simulink library "xbsStateMachine_r2"  (Simulink 5.0)
undefined symbols (not defined in the file or in its folder): xlDistRamDepth, xlMatrixToOutputVec, xlMatrixToStateInitVec, xlNumMealyElements, xlNumMooreOutputElements, xlNumMooreStateElements, xlNumStateBits, xlRegMealyInitVec
libraries: xbsMemory_r2 x7, xbsBasic_r2 x6
settings Model: Creator=administrator  LastModifiedBy=mcmillan

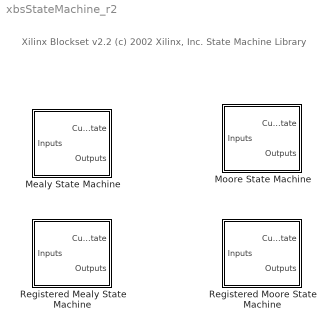
== system xbsStateMachine_r2 ==
  note: Xilinx Blockset v2.2
      | (c) 2002 Xilinx, Inc.
      |
      | State Machine Library
  Mealy State Machine : Subsystem  mask(Xilinx Mealy State Machine){next_state_matrix=[0 1; 2 1; 0 3; 2 1], output_matrix=[0 0; 0 0; 0 0; 0 1], n_bits=1, period=1, xl_area=[0, 0, 0, 0, 0, 0, 0], xl_use_area=off}
      mask prompts: next_state_matrix "Next State Matrix"; output_matrix "Output Matrix"; n_bits "Number of  Output Bits"; period "Sample Period"; xl_area "FPGA Area [Slices, FFs, BRAMs, LUTs, IOBs, Emb. Mults, TBUFs]"; xl_use_area "Use Area Above For Estimation"
      mask help: Implements a Mealy state machine. The output is a function of the current state and input.
      mask init:
      | % Set Block Logo
      | [bg,fg] = xlcmap('XBlock',0);
      | iPos = get_param(gcb,'Position');
      | iWidth=iPos(3)-iPos(1); iHeight=iPos(4)-iPos(2);
      | iCx=iWidth/2;
      | iCy=iHeight/2;
      | [logoX, logoY] = xlogo(iPos);
      mask Help: web(xldoclink('Mealy State Machine'));
      mask Display:
      | patch([0 iWidth iWidth 0],[0 0 iHeight iHeight] , bg);
      | patch(logoX,logoY, fg);
      | port_label('input',1,'Inputs');
      | port_label('output',1,'CurrentState');
      | port_label('output',2,'Outputs');
      | 
      | plot([0 0 iWidth iWidth 0], [0 iHeight iHeight 0 0]);
  Moore State Machine : Subsystem  mask(Xilinx Moore State Machine){next_state_matrix=[0 1; 2 1; 0 3; 2 4; 0 1], output_matrix=[0; 0; 0; 0; 1], n_bits=1, period=1, xl_area=[0, 0, 0, 0, 0, 0, 0], xl_use_area=off}
      mask prompts: next_state_matrix "Next State Matrix"; output_matrix "Output Array"; n_bits "Number of Output Bits"; period "Sample Period"; xl_area "FPGA Area [Slices, FFs, BRAMs, LUTs, IOBs, Emb. Mults, TBUFs]"; xl_use_area "Use Area Above For Estimation"
      mask help: Implements a Moore state machine. The output is a function only of the current state.
      mask init:
      | % Set Block Logo
      | [bg,fg] = xlcmap('XBlock',0);
      | iPos = get_param(gcb,'Position');
      | iWidth=iPos(3)-iPos(1); iHeight=iPos(4)-iPos(2);
      | iCx=iWidth/2;
      | iCy=iHeight/2;
      | [logoX, logoY] = xlogo(iPos);
      mask Help: web(xldoclink('Moore State Machine'));
      mask Display:
      | patch([0 iWidth iWidth 0],[0 0 iHeight iHeight] , bg);
      | patch(logoX,logoY, fg);
      | port_label('input',1,'Inputs');
      | port_label('output',1,'CurrentState');
      | port_label('output',2,'Outputs');
      | 
      | plot([0 0 iWidth iWidth 0], [0 iHeight iHeight 0 0]);
  Registered Mealy State Machine : Subsystem  mask(Xilinx Registered Mealy State Machine){next_state_matrix=[0 1; 2 1; 0 3; 2 1], output_matrix=[0 0; 0 0; 0 0; 0 1], n_bits=1, period=1, xl_area=[0, 0, 0, 0, 0, 0, 0], xl_use_area=off}
      mask prompts: next_state_matrix "Next State Matrix"; output_matrix "Output Matrix"; n_bits "Number of Output Bits"; period "Sample Period"; xl_area "FPGA Area [Slices, FFs, BRAMs, LUTs, IOBs, Emb. Mults, TBUFs]"; xl_use_area "Use Area Above For Estimation"
      mask help: Implements a registered Mealy state machine. The output is a function of the current state and its input. The output is registered.
      mask init:
      | % Set Block Logo
      | [bg,fg] = xlcmap('XBlock',0);
      | iPos = get_param(gcb,'Position');
      | iWidth=iPos(3)-iPos(1); iHeight=iPos(4)-iPos(2);
      | iCx=iWidth/2;
      | iCy=iHeight/2;
      | [logoX, logoY] = xlogo(iPos);
      mask Help: web(xldoclink('Registered Mealy State Machine'));
      mask Display:
      | patch([0 iWidth iWidth 0],[0 0 iHeight iHeight] , bg);
      | patch(logoX,logoY, fg);
      | port_label('input',1,'Inputs');
      | port_label('output',1,'CurrentState');
      | port_label('output',2,'Outputs');
      | 
      | plot([0 0 iWidth iWidth 0], [0 iHeight iHeight 0 0]);
  Registered Moore State Machine : Subsystem  mask(Xilinx Registered Moore State Machine){next_state_matrix=[0 1; 2 1; 0 3; 2 4; 0 1], output_matrix=[0; 0; 0; 0; 1], n_bits=1, period=1, xl_area=[0, 0, 0, 0, 0, 0, 0], xl_use_area=off}
      mask prompts: next_state_matrix "Next State Matrix"; output_matrix "Output Array"; n_bits "Number of Output Bits"; period "Sample Period"; xl_area "FPGA Area [Slices, FFs, BRAMs, LUTs, IOBs, Emb. Mults, TBUFs]"; xl_use_area "Use Area Above For Estimation"
      mask help: Implements a registered Moore state machine. The output is a function only of the current state. The output is registered.
      mask init:
      | % Set Block Logo
      | [bg,fg] = xlcmap('XBlock',0);
      | iPos = get_param(gcb,'Position');
      | iWidth=iPos(3)-iPos(1); iHeight=iPos(4)-iPos(2);
      | iCx=iWidth/2;
      | iCy=iHeight/2;
      | [logoX, logoY] = xlogo(iPos);
      mask Help: web(xldoclink('Registered Moore State Machine'));
      mask Display:
      | patch([0 iWidth iWidth 0],[0 0 iHeight iHeight] , bg);
      | patch(logoX,logoY, fg);
      | port_label('input',1,'Inputs');
      | port_label('output',1,'CurrentState');
      | port_label('output',2,'Outputs');
      | 
      | plot([0 0 iWidth iWidth 0], [0 iHeight iHeight 0 0]);

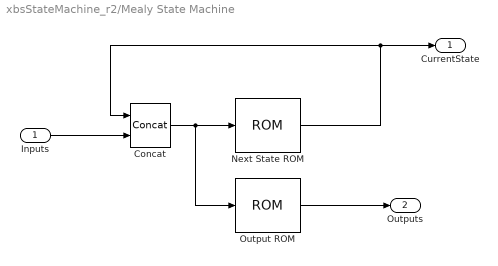
== system xbsStateMachine_r2/Mealy State Machine ==
  Inputs : Inport
  Concat : xbsBasic_r2/Concat  explicit_period=off  period=1  trim_vbits=off  dbl_ovrd=off
  Next State ROM : xbsMemory_r2/ROM  depth=xlNumMealyElements(next_state_matrix, output_matrix)  initVector=xlMatrixToStateInitVec(next_state_matrix,xlNumStateBits(next_state_matrix),0,1,1,1)  arith_type=Unsigned  n_bits=xlNumStateBits(next_state_matrix)  bin_pt=0  init_zero=on  latency=1  explicit_period=on  period=period  en=off  trim_vbits=off  dbl_ovrd=off  distributed_mem=off  gen_core=on  use_rpm=off
  Output ROM : xbsMemory_r2/ROM  depth=xlDistRamDepth(output_matrix)  initVector=xlMatrixToOutputVec(output_matrix,n_bits,0,1,1,1)  arith_type=Unsigned  n_bits=n_bits  bin_pt=0  init_zero=on  latency=0  explicit_period=on  period=period  en=off  trim_vbits=off  dbl_ovrd=off  distributed_mem=on  gen_core=on  use_rpm=off
  CurrentState : Outport
  Outputs : Outport  Port=2
  wires:
  Inputs/1 -> Concat/2
  Output ROM/1 -> Outputs/1
  Concat/1 -> Next State ROM/1, Output ROM/1
  Next State ROM/1 -> Concat/1, CurrentState/1

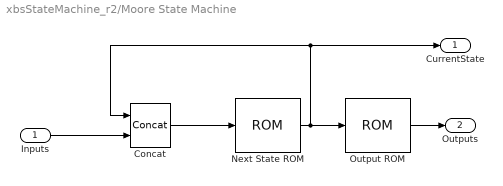
== system xbsStateMachine_r2/Moore State Machine ==
  Inputs : Inport
  Concat : xbsBasic_r2/Concat  explicit_period=off  period=1  trim_vbits=off  dbl_ovrd=off
  Next State ROM : xbsMemory_r2/ROM  depth=xlNumMooreStateElements(next_state_matrix, output_matrix)  initVector=xlMatrixToStateInitVec(next_state_matrix,xlNumStateBits(next_state_matrix),0,1,1,1)  arith_type=Unsigned  n_bits=xlNumStateBits(next_state_matrix)  bin_pt=0  init_zero=on  latency=1  explicit_period=on  period=period  en=off  trim_vbits=off  dbl_ovrd=off  distributed_mem=off  gen_core=on  use_rpm=off
  Output ROM : xbsMemory_r2/ROM  depth=xlDistRamDepth(output_matrix)  initVector=xlMatrixToOutputVec(output_matrix,n_bits,0,1,1,1)  arith_type=Unsigned  n_bits=n_bits  bin_pt=0  init_zero=on  latency=0  explicit_period=on  period=period  en=off  trim_vbits=off  dbl_ovrd=off  distributed_mem=on  gen_core=on  use_rpm=off
  CurrentState : Outport
  Outputs : Outport  Port=2
  wires:
  Inputs/1 -> Concat/2
  Output ROM/1 -> Outputs/1
  Concat/1 -> Next State ROM/1
  Next State ROM/1 -> Concat/1, CurrentState/1, Output ROM/1

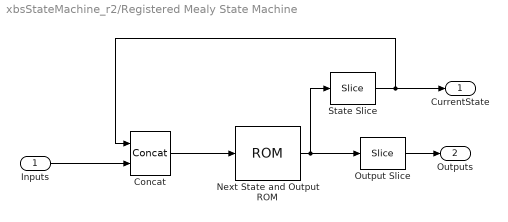
== system xbsStateMachine_r2/Registered Mealy State Machine ==
  Inputs : Inport
  Concat : xbsBasic_r2/Concat  explicit_period=off  period=1  trim_vbits=off  dbl_ovrd=off
  Next State and Output ROM : xbsMemory_r2/ROM  depth=xlNumMealyElements(next_state_matrix, output_matrix)  initVector=xlRegMealyInitVec(next_state_matrix, output_matrix, n_bits,0,1,1,1)  arith_type=Unsigned  n_bits=xlNumStateBits(next_state_matrix)+n_bits  bin_pt=0  init_zero=on  latency=1  explicit_period=on  period=period  en=off  trim_vbits=off  dbl_ovrd=off  distributed_mem=off  gen_core=on  use_rpm=off
  Output Slice : xbsBasic_r2/Slice  mode=Lower Bit Location + Width  nbits=n_bits  bit1=0  base1=MSB of Input  bit0=0  base0=LSB of Input  boolean_output=off  explicit_period=off  period=1  trim_vbits=off  dbl_ovrd=off
  State Slice : xbsBasic_r2/Slice  mode=Upper Bit Location + Width  nbits=xlNumStateBits(next_state_matrix)  bit1=0  base1=MSB of Input  bit0=0  base0=LSB of Input  boolean_output=off  explicit_period=off  period=1  trim_vbits=off  dbl_ovrd=off
  CurrentState : Outport
  Outputs : Outport  Port=2
  wires:
  Inputs/1 -> Concat/2
  Output Slice/1 -> Outputs/1
  Concat/1 -> Next State and Output ROM/1
  Next State and Output ROM/1 -> Output Slice/1, State Slice/1
  State Slice/1 -> CurrentState/1, Concat/1

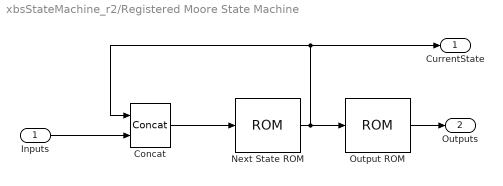
== system xbsStateMachine_r2/Registered Moore State Machine ==
  Inputs : Inport
  Concat : xbsBasic_r2/Concat  explicit_period=off  period=1  trim_vbits=off  dbl_ovrd=off
  Next State ROM : xbsMemory_r2/ROM  depth=xlNumMooreStateElements(next_state_matrix, output_matrix)  initVector=xlMatrixToStateInitVec(next_state_matrix,xlNumStateBits(next_state_matrix),0,1,1,1)  arith_type=Unsigned  n_bits=xlNumStateBits(next_state_matrix)  bin_pt=0  init_zero=on  latency=1  explicit_period=on  period=period  en=off  trim_vbits=off  dbl_ovrd=off  distributed_mem=off  gen_core=on  use_rpm=off
  Output ROM : xbsMemory_r2/ROM  depth=xlNumMooreOutputElements(output_matrix)  initVector=xlMatrixToOutputVec(output_matrix,n_bits,0,1,1,1)  arith_type=Unsigned  n_bits=n_bits  bin_pt=0  init_zero=on  latency=1  explicit_period=on  period=period  en=off  trim_vbits=off  dbl_ovrd=off  distributed_mem=off  gen_core=on  use_rpm=off
  CurrentState : Outport
  Outputs : Outport  Port=2
  wires:
  Next State ROM/1 -> Output ROM/1, CurrentState/1, Concat/1
  Concat/1 -> Next State ROM/1
  Output ROM/1 -> Outputs/1
  Inputs/1 -> Concat/2
